simulink model "moban1"  (R2022b)
settings: Solver=VariableStepAuto  StartTime=0.0  StopTime=4  RelTol=1e-3
InitFcn:
  | clear all;
  | 
  | Step_time=2;  %并网转离网的切换时间
  | Tf=0.0159*0.25 %直流侧电流滤波常数
  | 
  | Vdc_H2=720;   %直流母线电压最大值
  | Vdc_H1=710;   %
  | Udc=700;   %直流母线电压最大值
  | Vdc_L1=690;
  | Vdc_L2=680;   %直流母线电压最小值
  | 
  | %% 并网变流器部分 %%
  | P_grid=100e3;  %变流器额定功率
  | Cg=3227e-6;   %直流母线电容
  | P_grid=100e3;  %变流器额定功率
  | Idc_max=145;   %直流侧最大输出电流
  | %Rg=(720-700)/Idc_max;   %下垂系数
  | Rg=40*(Udc-40)/P_grid;   %下垂系数
  | Igrid_max=72;   %并网逆变器最大充放电电流（交流侧）
  | 
  | %% 蓄电池部分 %%
  | P_ba=50e3;  %变流器额定功率
  | R_ba=40*(Udc-40)/P_ba;
  | %Idc_max_ba=147;   %直流侧最大输出电流
  | %R_ba=(Vdc_L1-Vdc_L2)/P_ba;   %下垂系数
  | Iba_max=50;   %蓄电池恒流充放电电流
  | 
  | %% 光伏部分 %%
  | P_PV=150e3;  %变流器额定功率
  | R_PV=40*(Udc-40)/P_PV;   %下垂系数
  | Idc_max_PV=147;   %直流侧最大输出电流
model workspace (MAT data in the model file):
  C = 0.002
  GP = 1
  GQ = 0.01
  J = 5
  KQ = 0.06
  Kf = 800
  Kv = 577
  L = 0.002
  Ts = 5e-05
  Vdc = 400
  fsw = 20000
  wn = 314.159265359
undefined symbols (not defined in the file): DiscIntNeverNeededParam, Ion, Lithium, sigbuilder_block
libraries: spsCurrentMeasurementLib x8, spsSeriesRLCBranchLib x6, slpidlib x6, spsDiodeLib x4, spsVoltageMeasurementLib x3, spsFirstOrderFilterLib x3, spsabctodq0Lib x3, spsIGBTLib x3, spsThreePhaseSeriesRLCBranchLib x2, spsThreePhaseVIMeasurementLib x2, simulink x2, spsPower3phInstantaneousLib x1
(part 2 of 2)

== system moban1/电池模块/Subsystem/Subsystem2 ==
  In1 : Inport
  Constant1 : Constant
  Constant2 : Constant  Value=0
  Repeating Sequence : simulink/Sources/Repeating Sequence  rep_seq_t=[0 0.00005 0.0001]  rep_seq_y=[-1 1 -1]
  Saturation1 : Saturate  UpperLimit=1  LowerLimit=-1
  Subtract2 : Sum  Inputs=+-
  Switch : Switch  SaturateOnIntegerOverflow=off  InputSameDT=off
  Out1 : Outport  VectorParamsAs1DForOutWhenUnconnected=off
  wires:
  Switch/1 -> Out1/1
  Constant2/1 -> Switch/3
  Constant1/1 -> Switch/1
  Repeating Sequence/1 -> Subtract2/2
  Subtract2/1 -> Switch/2
  Saturation1/1 -> Subtract2/1
  In1/1 -> Saturation1/1
